simulink model "controlSystem_TorqueOptimizer"  (R2021a)
settings: Solver=VariableStepAuto  StartTime=0.0  StopTime=30  RelTol=1e-7
values from neighbouring files (symbols this model uses):
  initialFuel = 100    [data.m]
  maxEngineTemp = 240    [data.m]
  maxEngineTorque = 80    [data.m]
  maxMotorTemp = 135    [data.m]
  maxMotorTorque = 80    [data.m]
  maxRegenTorque = 80    [data.m]
  motorVoltage = 140    [data.m]
undefined symbols (not defined in the file or in its folder): sigbuilder_block
libraries: autolibshared x4, autolibsharedcoupling x3, autolibhevctrlrcommon x2, autolibmappedmotor x2, autolibshareddiff x1, autolibtransamt x1, autolibdcdc x1, autolibdatasheetbattery x1, autolibsharedmappedengines x1
(part 1 of 5)
settings Model: Creator=peter  LastModifiedBy=peter
settings DebuggingCC: SFMachineParentedDataDiag=warning

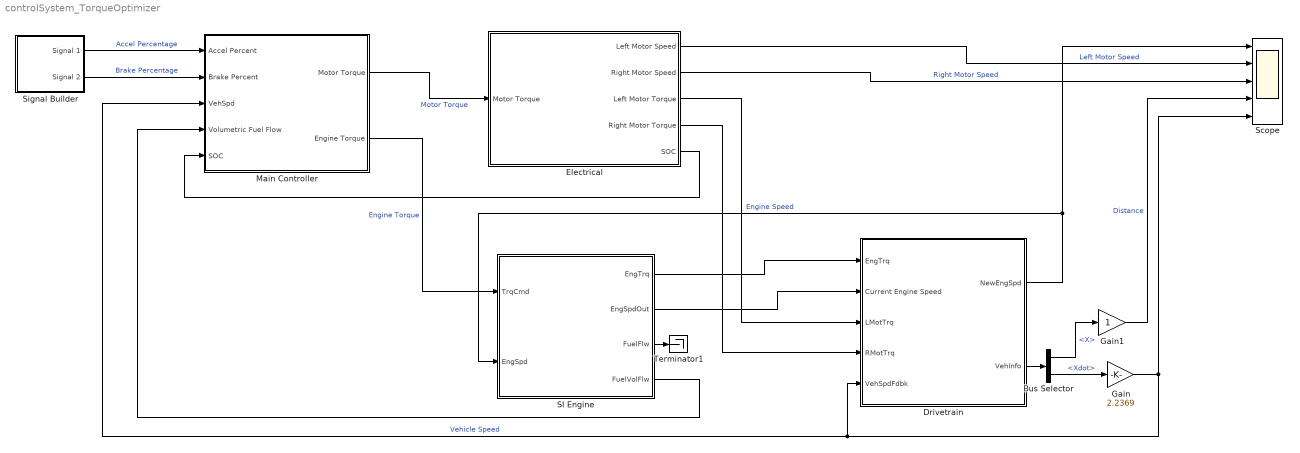
== system controlSystem_TorqueOptimizer ==
  Bus Selector : BusSelector  OutputSignals=InertFrm.Cg.Disp.X,InertFrm.Cg.Vel.Xdot
  Drivetrain : Subsystem
  Electrical : Subsystem
  Gain : Gain  Gain=2.2369
  Gain1 : Gain
  Main Controller : Subsystem
  SI Engine : Subsystem
  Scope : Scope  NumInputPorts=5
  Signal Builder : Subsystem  Tag=STV Subsys  LoadFcn=sigbuilder_block('load');  StartFcn=sigbuilder_block('start');  StopFcn=sigbuilder_block('stop');  ClipboardFcn=sigbuilder_block('clipboard');  mask(Sigbuilder block){tuvar=[0:10]}
      mask help: Simulink:masks:SigbuilderBlock_MD
      mask init:
      | if ~strcmp(get_param(bdroot(gcbh),'SimulationStatus'),'stopped') tuvar = sigbuilder_block('maskInit'); end
      settings: CopyFcn=sigbuilder_block('copy');  DeleteFcn=sigbuilder_block('delete');  ModelCloseFcn=sigbuilder_block('modelClose');  PreSaveFcn=sigbuilder_block('preSave');  PauseFcn=sigbuilder_block('pause');  ContinueFcn=sigbuilder_block('continue');  NameChangeFcn=sigbuilder_block('namechange');  OpenFcn=sigbuilder_block('open',[334.2 75 550.8 400.2 ]);  CloseFcn=sigbuilder_block('close');
      mask Display: plot(0, 0, 100, 100,[2, 2, 32, 32, 2], [68, 8, 8, 68, 68],[32, 2], [38, 38], [32, 19, 2],[53, 60, 44], [32, 17, 17, 2],[16, 16, 31, 31]);txt = getActiveGroup(gcbh);text(2, 100, txt,'verticalAlignment', 'top');
  Terminator1 : Terminator
  wires:
  Signal Builder/1(Signal 1) -> Main Controller/1(Accel Percent)  "Accel Percentage"
  Electrical/5(SOC) -> Main Controller/5(SOC)
  Signal Builder/2(Signal 2) -> Main Controller/2(Brake Percent)  "Brake Percentage"
  Main Controller/1(Motor Torque) -> Electrical/1(Motor Torque)  "Motor Torque"
  Main Controller/2(Engine Torque) -> SI Engine/1(TrqCmd)  "Engine Torque"
  Drivetrain/1(NewEngSpd) -> Scope/1, SI Engine/2(EngSpd)  "Engine Speed"
  SI Engine/3(FuelFlw) -> Terminator1/1
  SI Engine/4(FuelVolFlw) -> Main Controller/4(Volumetric Fuel Flow)
  SI Engine/2(EngSpdOut) -> Drivetrain/2(Current Engine Speed)
  SI Engine/1(EngTrq) -> Drivetrain/1(EngTrq)
  Electrical/3(Left Motor Torque) -> Drivetrain/3(LMotTrq)
  Electrical/4(Right Motor Torque) -> Drivetrain/4(RMotTrq)
  Electrical/1(Left Motor Speed) -> Scope/2  "Left Motor Speed"
  Electrical/2(Right Motor Speed) -> Scope/3  "Right Motor Speed"
  Drivetrain/2(VehInfo) -> Bus Selector/1
  Bus Selector/1 -> Gain1/1  "<X>"
  Bus Selector/2 -> Gain/1  "<Xdot>"
  Gain/1 -> Scope/5, Main Controller/3(VehSpd), Drivetrain/5(VehSpdFdbk)  "Vehicle Speed"
  Gain1/1 -> Scope/4  "Distance"

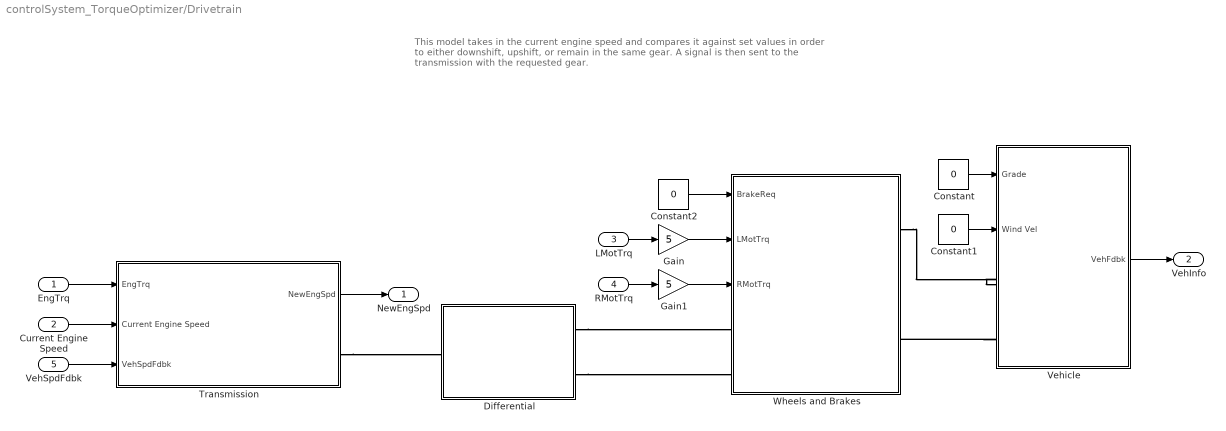
== system controlSystem_TorqueOptimizer/Drivetrain ==
  note: This model takes in the current engine speed and compares it against set values in order to either downshift, upshift, or remain in the same gear. A signal is then sent to the transmission with the requested gear.
  EngTrq : Inport
  Current Engine Speed : Inport  Port=2
  LMotTrq : Inport  Port=3
  RMotTrq : Inport  Port=4
  VehSpdFdbk : Inport  Port=5
  Constant : Constant  Value=0
  Constant1 : Constant  Value=0
  Constant2 : Constant  Value=0
  Differential : Subsystem
  Gain : Gain  Gain=5
  Gain1 : Gain  Gain=5
  Transmission : Subsystem
  Vehicle : Subsystem
  Wheels and Brakes : Subsystem  VariantControl=0
  NewEngSpd : Outport
  VehInfo : Outport  Port=2
  wires:
  Constant/1 -> Vehicle/1(Grade)
  Constant1/1 -> Vehicle/2(Wind Vel)
  Constant2/1 -> Wheels and Brakes/1(BrakeReq)
  EngTrq/1 -> Transmission/1(EngTrq)
  Current Engine Speed/1 -> Transmission/2(Current Engine Speed)
  VehSpdFdbk/1 -> Transmission/3(VehSpdFdbk)
  Transmission/1(NewEngSpd) -> NewEngSpd/1
  Vehicle/1(VehFdbk) -> VehInfo/1
  LMotTrq/1 -> Gain/1
  RMotTrq/1 -> Gain1/1
  Gain/1 -> Wheels and Brakes/2(LMotTrq)
  Gain1/1 -> Wheels and Brakes/3(RMotTrq)
  connections:
  Wheels and Brakes/RConn1 -- Vehicle/LConn1
  Vehicle/LConn2 -- Wheels and Brakes/RConn2
  Transmission/RConn1 -- Differential/LConn1
  Differential/RConn1 -- Wheels and Brakes/LConn1
  Differential/RConn2 -- Wheels and Brakes/LConn2

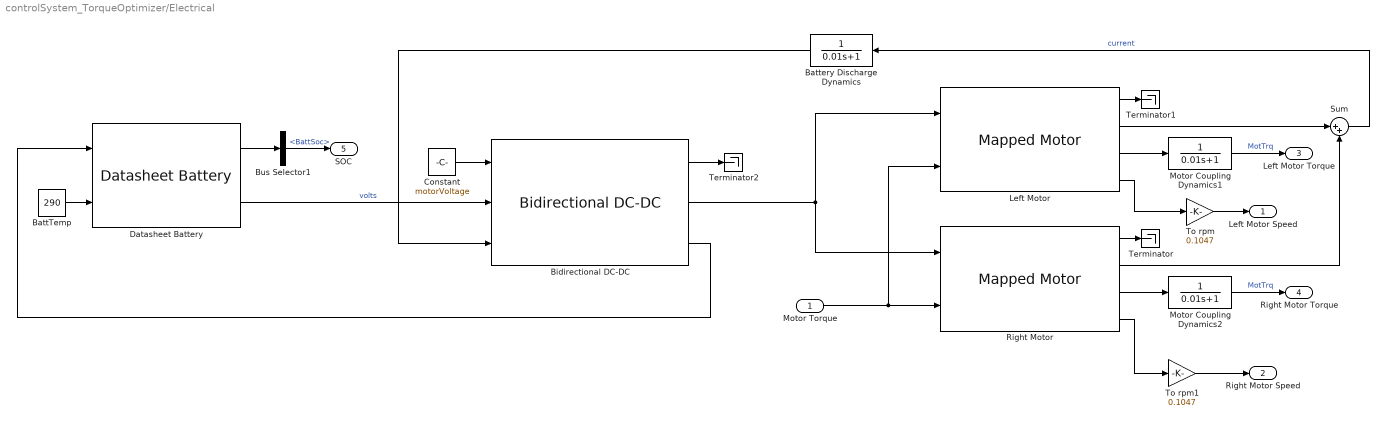
== system controlSystem_TorqueOptimizer/Electrical ==
  Motor Torque : Inport
  " Right Motor" : autolibmappedmotor/Mapped Motor  port_config=Torque  param_by=Tabulated torque-speed envelope  w_t=motorSpeeds  T_t=motorTorques  power_max=30000  Tc=0.02  param_loss=Single efficiency measurement  eff=100  w_eff=375  T_eff=0.08  Piron=0  Pbase=0  w_eff_bp=[-8000 -4000 0 4000 8000]  T_eff_bp=[0 0.03 0.06 0.09]  Temp_eff_bp=[233.15 293.15 373.15]  losses_table=[1.49 1.67 2.21 3.10; 0.42 0.69 1.14 2.03; 0.06 0.24 0.78 1.68; 0.42 0.69 1.14 2.03; 1.49 1.67 2.21 3.10]  losses_table_3d=cat(3,1.05*[1.49 1.67 2.21 3.10; 0.42 0.69 1.14 2.03; 0.06 0.24 0.78 1.68; 0.42 0.69 1.14 2.03; 1.49 1.67 2.21 3.10],[1.49 1.67 2.21 3.10; 0.42 0.69 1.14 2.03; 0.06 0.24 0.78 1.68; 0.42 0.69 1.14 2.03; 1.49 1.67 2.21 3.10],1.03*[1.49 1.67 2.21 3.10; 0.42 0.69 1.14 2.03; 0.06 0.24 0.78 1.68; 0.42 0.69 1.14 2.03; 1.49 1.67 2.21 3.10])  efficiency_table=[95 95 95 95; 95 95 95 95; 95 95 95 95; 95 95 95 95; 95 95 95 95]  efficiency_table_3d=cat(3,90*ones(5,4),95*ones(5,4),92*ones(5,4))  J=5e-6  b=1e-5  omega_o=0  T_t_extended=[80 80 80 80 80 80 80 80 80 80 80 80 80 80 80]  w_t_extended=[-733.061053513457 -628.338045868677 -523.615038223898 -418.892030579118 -314.169022934339 -209.446015289559 -104.72300764478 0 104.72300764478 209.446015289559 314.169022934339 418.892030579118 523.615038223898 628.338045868677 733.061053513457]  KLossIron=0  KLossCopper=0  x_w_eff_vec=[-8000 -4000 0 4000 8000]  x_T_eff_vec=[-0.09 -0.06 -0.03 0 0.03 0.06 0.09]  x_tmp_eff_vec=[233.15 293.15 373.15]  x_losses_mat=[3.1 2.21 1.67 1.49 1.67 2.21 3.1;2.03 1.14 0.69 0.42 0.69 1.14 2.03;1.68 0.78 0.24 0.06 0.24 0.78 1.68;2.03 1.14 0.69 0.42 0.69 1.14 2.03;3.1 2.21 1.67 1.49 1.67 2.21 3.1]  x_losses_mat_3d=cat(3,[3.255 2.3205 1.7535 1.5645 1.7535 2.3205 3.255;2.1315 1.197 0.7245 0.441 0.7245 1.197 2.1315;1.764 0.819 0.252 0.063 0.252 0.819 1.764;2.1315 1.197 0.7245 0.441 0.7245 1.197 2.1315;3.255 2.3205 1.7535 1.5645 1.7535 2.3205 3.255],[3.1 2.21 1.67 1.49 1.67 2.21 3.1;2.03 1.14 0.69 0.42 0.69 1.14 2.03;1.68 0.78 0.24 0.06 0.24 0.78 1.68;2.03 1.14 0.69 0.42 0.69 1.14 2.03;3.1 2.21 1.67 1.49 1.67 2.21 3.1],[3.193 2.2763 1.7201 1.5347 1.7201 2.2763 3.193;2.0909 1.1742 0.7107 0.4326 0.7107 1.1742 2.0909;1.7304 0.8034 0.2472 0.0618 0.2472 0.8034 1.7304;2.0909 1.1742 0.7107 0.4326 0.7107 1.1742 2.0909;3.193 2.2763 1.7201 1.5347 1.7201 2.2763 3.193])  CalLossMapData={}  CalLossWithTempMapData={}  aMode=2  RefBlkName='autolibmappedmotor/Mapped Motor'
      settings: SourceProductBaseCode=PW,DR,MT,UV,VE
  BattTemp : Constant  Value=290
  Battery Discharge Dynamics : TransferFcn  Denominator=[0.01 1]
  Bidirectional DC-DC : autolibdcdc/Bidirectional DC-DC  Tc=1/1000  Vinit=0  Plimit=100000  param_loss=Single efficiency measurement  eff=98  v_loss_bp=[0 200 400 600 800 1000]  i_loss_bp=[0 25 50 75 100]  losses_table=[100 100 100 100 100;100 150 200 250 300;100 200 300 400 500;100 250 400 550 700;100 300 500 700 900;100 350 600 850 1100]  v_eff_bp=[200 400 600 800 1000]  i_eff_bp=[25 50 75 100]  efficiency_table=[96.2 98.1 98.7 99;98.1 99 99.4 99.5;98.7 99.4 99.6 99.7;99 99.5 99.7 99.8;99.2 99.6 99.7 99.8]  x_v_bp=[-1000 -800 -600 -400 -200 200 400 600 800 1000]  x_i_bp=[-100 -75 -50 -25 25 50 75 100]  x_losses_mat=[200.400801603196 225.67703109328 200.803212851408 201.612903225806 199.999999999997 200 225 200;160.320641282556 180.541624874624 201.005025125625 202.020202020203 200 200 180 160;180.541624874624 180.722891566267 181.086519114686 197.568389057748 194.999999999999 179.999999999997 180 180;201.005025125625 181.086519114686 202.020202020203 193.67991845056 190 200 179.999999999997 200;202.020202020203 197.568389057748 193.67991845056 197.505197505197 190 190 194.999999999999 200;200 194.999999999999 190 190 197.505197505197 193.67991845056 197.568389057748 202.020202020203;200 179.999999999997 200 190 193.67991845056 202.020202020203 181.086519114686 201.005025125625;180 180 179.999999999997 194.999999999999 197.568389057748 181.086519114686 180.722891566267 180.541624874624;160 180 200 200 202.020202020203 201.005025125625 180.541624874624 160.320641282556;200 225 200 199.999999999997 201.612903225806 200.803212851408 225.67703109328 200.400801603196]  RefBlkName='autolibdcdc/Bidirectional DC-DC'
      settings: SourceProductBaseCode=PW
  Bus Selector1 : BusSelector  OutputSignals=BattSoc
  Constant : Constant  Value=motorVoltage
  Datasheet Battery : autolibdatasheetbattery/Datasheet Battery  CapacityCtrl=Parameter  OutputVlt=Unfiltered  BattChargeMax=100  Em=[2.8 3.228 3.284 3.361 3.408 3.427 3.472 3.477 3.493 3.504 3.516 3.528 3.537 3.545 3.555 3.561 3.566 3.576 3.587 3.589 3.594 3.6 3.608 3.61 3.616 3.619 3.626 3.632 3.637 3.64 3.645 3.646 3.652 3.655 3.658 3.661 3.664 3.668 3.673 3.678 3.68 3.681 3.686 3.692 3.699 3.702 3.705 3.71 3.717 3.723 3.728 3.733 3.735 3.742 3.749 3.755 3.761 3.768 3.773 3.78 3.791 3.798 3.798 3.814 3.818 3.825 3.841 3.846 3.855 3.863 3.877 3.885 3.894 3.907 3.919 3.926 3.935 3.944 3.954 3.964 3.974 3.988 3.998 4.014 4.029 4.034 4.047 4.065 4.074 4.086 4.097 4.131 4.126 4.138 4.15 4.18 4.174 4.187 4.207 4.231 4.221]  CapLUTBp=[0 0.01 0.02 0.03 0.04 0.05 0.06 0.07 0.08 0.09 0.1 0.11 0.12 0.13 0.14 0.15 0.16 0.17 0.18 0.19 0.2 0.21 0.22 0.23 0.24 0.25 0.26 0.27 0.28 0.29 0.3 0.31 0.32 0.33 0.34 0.35 0.36 0.37 0.38 0.39 0.4 0.41 0.42 0.43 0.44 0.45 0.46 0.47 0.48 0.49 0.5 0.51 0.52 0.53 0.54 0.55 0.56 0.57 0.58 0.59 0.6 0.61 0.62 0.63 0.64 0.65 0.66 0.67 0.68 0.69 0.7 0.71 0.72 0.73 0.74 0.75 0.76 0.77 0.78 0.79 0.8 0.81 0.82 0.83 0.84 0.85 0.86 0.87 0.88 0.89 0.9 0.91 0.92 0.93 0.94 0.95 0.96 0.97 0.98 0.99 1]  RInt=[0.008846 0.009319 0.009027 0.00847 0.01032 0.01314;0.006389 0.006554 0.005553 0.005525 0.006043 0.007805;0.004364 0.004101 0.00406 0.003452 0.003846 0.004517;0.002031 0.002563 0.002532 0.00246 0.002716 0.003047;0.001443 0.001825 0.001795 0.001778 0.001924 0.002234;0.0005603 0.0007192 0.0006887 0.0007557 0.0007355 0.001014;0.001028 0.001338 0.001 0.001536 0.001546 0.002789]  BattTempBp=[243.1 253.1 263.1 273.1 283.1 298.1 313.1]  CapSOCBp=[0 0.2 0.4 0.6 0.8 1]  Ns=32  Np=9  BattCapInit=100  Tc=1/1000  Vinit=4.221  RefBlkName='autolibdatasheetbattery/Datasheet Battery'
      settings: SourceProductBaseCode=PW
  Left Motor : autolibmappedmotor/Mapped Motor  port_config=Torque  param_by=Tabulated torque-speed envelope  w_t=motorSpeeds  T_t=motorTorques  torque_max=80  power_max=30000  Tc=0.02  param_loss=Single efficiency measurement  eff=100  w_eff=375  T_eff=0.08  Piron=0  Pbase=0  w_eff_bp=[-8000 -4000 0 4000 8000]  T_eff_bp=[0 0.03 0.06 0.09]  Temp_eff_bp=[233.15 293.15 373.15]  losses_table=[1.49 1.67 2.21 3.10; 0.42 0.69 1.14 2.03; 0.06 0.24 0.78 1.68; 0.42 0.69 1.14 2.03; 1.49 1.67 2.21 3.10]  losses_table_3d=cat(3,1.05*[1.49 1.67 2.21 3.10; 0.42 0.69 1.14 2.03; 0.06 0.24 0.78 1.68; 0.42 0.69 1.14 2.03; 1.49 1.67 2.21 3.10],[1.49 1.67 2.21 3.10; 0.42 0.69 1.14 2.03; 0.06 0.24 0.78 1.68; 0.42 0.69 1.14 2.03; 1.49 1.67 2.21 3.10],1.03*[1.49 1.67 2.21 3.10; 0.42 0.69 1.14 2.03; 0.06 0.24 0.78 1.68; 0.42 0.69 1.14 2.03; 1.49 1.67 2.21 3.10])  efficiency_table=[95 95 95 95; 95 95 95 95; 95 95 95 95; 95 95 95 95; 95 95 95 95]  efficiency_table_3d=cat(3,90*ones(5,4),95*ones(5,4),92*ones(5,4))  J=5e-6  b=1e-5  omega_o=0  T_t_extended=[80 80 80 80 80 80 80 80 80 80 80 80 80 80 80]  w_t_extended=[-733.061053513457 -628.338045868677 -523.615038223898 -418.892030579118 -314.169022934339 -209.446015289559 -104.72300764478 0 104.72300764478 209.446015289559 314.169022934339 418.892030579118 523.615038223898 628.338045868677 733.061053513457]  KLossIron=0  KLossCopper=0  x_w_eff_vec=[-8000 -4000 0 4000 8000]  x_T_eff_vec=[-0.09 -0.06 -0.03 0 0.03 0.06 0.09]  x_tmp_eff_vec=[233.15 293.15 373.15]  x_losses_mat=[3.1 2.21 1.67 1.49 1.67 2.21 3.1;2.03 1.14 0.69 0.42 0.69 1.14 2.03;1.68 0.78 0.24 0.06 0.24 0.78 1.68;2.03 1.14 0.69 0.42 0.69 1.14 2.03;3.1 2.21 1.67 1.49 1.67 2.21 3.1]  x_losses_mat_3d=cat(3,[3.255 2.3205 1.7535 1.5645 1.7535 2.3205 3.255;2.1315 1.197 0.7245 0.441 0.7245 1.197 2.1315;1.764 0.819 0.252 0.063 0.252 0.819 1.764;2.1315 1.197 0.7245 0.441 0.7245 1.197 2.1315;3.255 2.3205 1.7535 1.5645 1.7535 2.3205 3.255],[3.1 2.21 1.67 1.49 1.67 2.21 3.1;2.03 1.14 0.69 0.42 0.69 1.14 2.03;1.68 0.78 0.24 0.06 0.24 0.78 1.68;2.03 1.14 0.69 0.42 0.69 1.14 2.03;3.1 2.21 1.67 1.49 1.67 2.21 3.1],[3.193 2.2763 1.7201 1.5347 1.7201 2.2763 3.193;2.0909 1.1742 0.7107 0.4326 0.7107 1.1742 2.0909;1.7304 0.8034 0.2472 0.0618 0.2472 0.8034 1.7304;2.0909 1.1742 0.7107 0.4326 0.7107 1.1742 2.0909;3.193 2.2763 1.7201 1.5347 1.7201 2.2763 3.193])  CalLossMapData={}  CalLossWithTempMapData={}  aMode=2  RefBlkName='autolibmappedmotor/Mapped Motor'
      settings: SourceProductBaseCode=PW,DR,MT,UV,VE
  Motor Coupling Dynamics1 : TransferFcn  Denominator=[0.01 1]
  Motor Coupling Dynamics2 : TransferFcn  Denominator=[0.01 1]
  Sum : Sum  Inputs=|++
  Terminator : Terminator
  Terminator1 : Terminator
  Terminator2 : Terminator
  To rpm : Gain  Gain=0.1047
  To rpm1 : Gain  Gain=0.1047
  Left Motor Speed : Outport
  Right Motor Speed : Outport  Port=2
  Left Motor Torque : Outport  Port=3
  Right Motor Torque : Outport  Port=4
  SOC : Outport  Port=5
  wires:
  BattTemp/1 -> Datasheet Battery/2
  Datasheet Battery/1 -> Bus Selector1/1
  Left Motor/2 -> Sum/1
  " Right Motor"/4 -> To rpm1/1
  " Right Motor"/2 -> Sum/2
  Bus Selector1/1 -> SOC/1  "<BattSoc>"
  " Right Motor"/1 -> Terminator/1
  Left Motor/1 -> Terminator1/1
  Motor Torque/1 -> Left Motor/2, " Right Motor"/2
  Sum/1 -> Battery Discharge Dynamics/1  "current"
  Left Motor/3 -> Motor Coupling Dynamics1/1
  Motor Coupling Dynamics1/1 -> Left Motor Torque/1  "MotTrq"
  " Right Motor"/3 -> Motor Coupling Dynamics2/1
  Motor Coupling Dynamics2/1 -> Right Motor Torque/1  "MotTrq"
  Bidirectional DC-DC/2 -> Left Motor/1, " Right Motor"/1
  Datasheet Battery/2 -> Bidirectional DC-DC/2  "volts"
  Constant/1 -> Bidirectional DC-DC/1
  Bidirectional DC-DC/3 -> Datasheet Battery/1
  Battery Discharge Dynamics/1 -> Bidirectional DC-DC/3
  Bidirectional DC-DC/1 -> Terminator2/1
  To rpm1/1 -> Right Motor Speed/1
  Left Motor/4 -> To rpm/1
  To rpm/1 -> Left Motor Speed/1

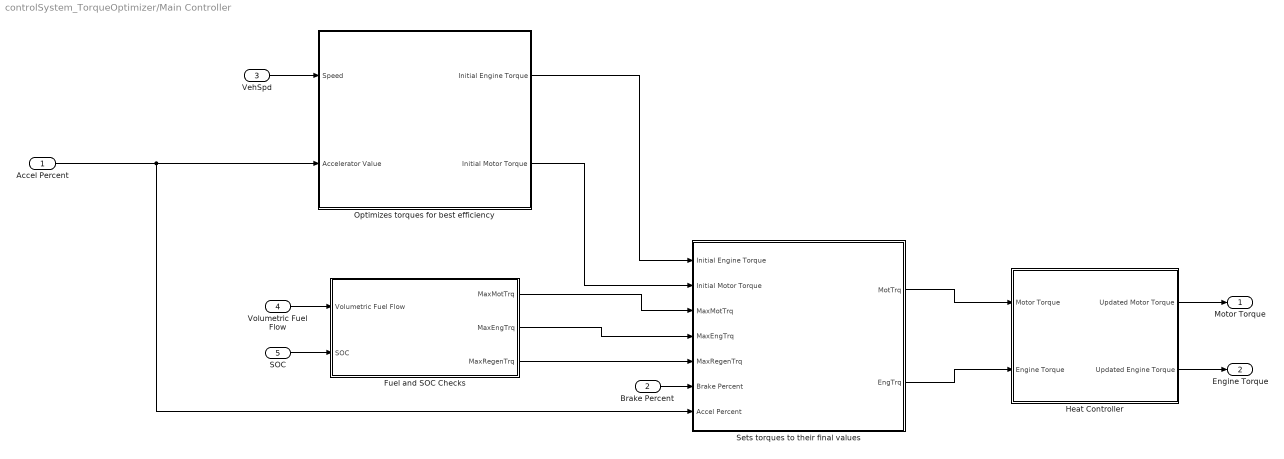
== system controlSystem_TorqueOptimizer/Main Controller ==
  Accel Percent : Inport
  Brake Percent : Inport  Port=2
  VehSpd : Inport  Port=3
  Volumetric Fuel Flow : Inport  Port=4
  SOC : Inport  Port=5
  Fuel and SOC Checks : Subsystem
  Heat Controller : Subsystem
  Optimizes torques for best efficiency : Subsystem
  Sets torques to their final values : Subsystem
  Motor Torque : Outport
  Engine Torque : Outport  Port=2
  wires:
  Accel Percent/1 -> Sets torques to their final values/7(Accel Percent), Optimizes torques for best efficiency/2(Accelerator Value)
  VehSpd/1 -> Optimizes torques for best efficiency/1(Speed)
  Volumetric Fuel Flow/1 -> Fuel and SOC Checks/1(Volumetric Fuel Flow)
  SOC/1 -> Fuel and SOC Checks/2(SOC)
  Heat Controller/1(Updated Motor Torque) -> Motor Torque/1
  Heat Controller/2(Updated Engine Torque) -> Engine Torque/1
  Optimizes torques for best efficiency/1(Initial Engine Torque) -> Sets torques to their final values/1(Initial Engine Torque)
  Optimizes torques for best efficiency/2(Initial Motor Torque) -> Sets torques to their final values/2(Initial Motor Torque)
  Fuel and SOC Checks/1(MaxMotTrq) -> Sets torques to their final values/3(MaxMotTrq)
  Fuel and SOC Checks/2(MaxEngTrq) -> Sets torques to their final values/4(MaxEngTrq)
  Fuel and SOC Checks/3(MaxRegenTrq) -> Sets torques to their final values/5(MaxRegenTrq)
  Brake Percent/1 -> Sets torques to their final values/6(Brake Percent)
  Sets torques to their final values/1(MotTrq) -> Heat Controller/1(Motor Torque)
  Sets torques to their final values/2(EngTrq) -> Heat Controller/2(Engine Torque)
